simulink model "ANDROID_MODEL"  (R2022b)
settings: Solver=FixedStepAuto  StartTime=0.0  StopTime=inf  RelTol=1e-3
libraries: androiduilib x5, androidcommunicationlib x5, visiongeotforms x3, visionanalysis x1, androidaudiovideolib x1
settings Model: Creator=VIKAS CHEIIURU  LastModifiedBy=VIKAS CHEIIURU
settings SolverCC: PositivePriorityOrder=on
settings OptimizationCC: EnhancedBackFolding=on  PassReuseOutputArgsAs=Individual arguments  ZeroExternalMemoryAtStartup=off  ZeroInternalMemoryAtStartup=off  MaxStackSize=64  OptimizeBlockOrder=speed  DifferentSizesBufferReuse=on  OptimizationCustomize=off  EfficientTunableParamExpr=on
settings DebuggingCC: ParameterTunabilityLossMsg=error
settings HardwareCC: ProdBitPerPointer=32  ProdBitPerSizeT=32  ProdBitPerPtrDiffT=32  ProdLargestAtomicInteger=Long  ProdLargestAtomicFloat=Double  ProdWordSize=32  ProdHWDeviceType=ARM Compatible->ARM Cortex
settings RTWCC: Description=Embedded Coder  SystemTargetFile=ert.tlc  HardwareBoard=Android Device  TLCOptions="-aInlineSetEventsForThisBaseRateFcn=TLC_FALSE -aSuppressMultiTaskScheduler=TLC_FALSE  -aRateBasedStepFcn=0"  TemplateMakefile=ert_default_tmf  RTWVerbose=off  Toolchain=Android SDK/NDK Tools  BuildConfiguration=Faster Runs
settings CodeAppCC: ForceParamTrailComments=on  IgnoreCustomStorageClasses=off  OperatorAnnotations=on  SimulinkDataObjDesc=on  SFDataObjDesc=on  InsertBlockDesc=on
settings ERTTargetCC: SupportVariableSizeSignals=on  ExtModeStaticAlloc=on

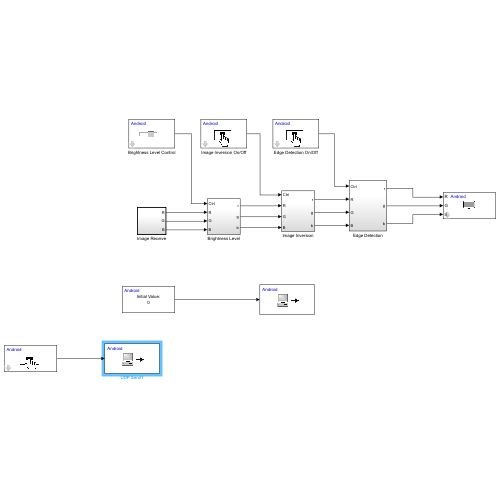
[thumbnail: Simulink's stored preview of the top-level diagram]
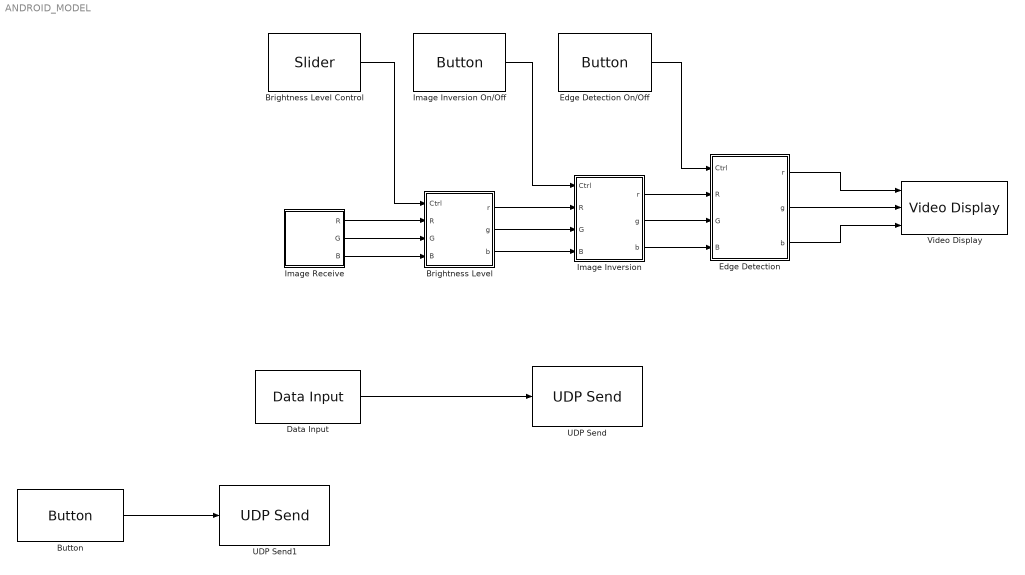
== system ANDROID_MODEL ==
  Brightness Level : Subsystem
  Brightness Level Control : androiduilib/Slider  Min=1  Value=1  Max=4  Resolution=0.1  SliderId=ANDROID_MODEL/Brightness_Level_Control  SampleTime=0.1  BlockPlatform=Android
  Button : androiduilib/Button  ButtonState=Not pressed  ButtonId=ANDROID_MODEL/Button  State=off  SampleTime=0.01  BlockPlatform=Android
  Data Input : androiduilib/Data Input  isCharVector=off  Value=0  CharVector=Hello World  OutputDataType=double  maxCharVectorSize=100  DataInputId=ANDROID_MODEL/Data_Input  SampleTime=0.01
  Edge Detection : Subsystem
  Edge Detection On/Off : androiduilib/Button  ButtonState=Not pressed  ButtonId=ANDROID_MODEL/Edge_Detection_On//Off  State=off  SampleTime=0.1  BlockPlatform=Android
  Image Inversion : Subsystem
  Image Inversion On/Off : androiduilib/Button  ButtonState=Not pressed  ButtonId=ANDROID_MODEL/Image_Inversion_On//Off  State=off  SampleTime=0.1  BlockPlatform=Android
  Image Receive : Subsystem  TreatAsAtomicUnit=on
  UDP Send : androidcommunicationlib/UDP Send  remoteURL='192.168.173.51'  remotePort=26001  localURL='0.0.0.0'  localPortSource=Automatically determine  localPort=-1  sampletime=-1  blockPlatform=Android  separateLengthPort=0
  UDP Send1 : androidcommunicationlib/UDP Send  remoteURL='192.168.173.51'  remotePort=26000  localURL='0.0.0.0'  localPortSource=Automatically determine  localPort=-1  sampletime=-1  blockPlatform=Android  separateLengthPort=0
  Video Display : androidaudiovideolib/Video Display  BlockPlatform=Android
  wires:
  Edge Detection/3(b) -> Video Display/3
  Brightness Level/2(g) -> Image Inversion/3(G)
  Image Inversion/3(b) -> Edge Detection/4(B)
  Image Receive/2(G) -> Brightness Level/3(G)
  Image Inversion On/Off/1 -> Image Inversion/1(Ctrl)
  Edge Detection On/Off/1 -> Edge Detection/1(Ctrl)
  Data Input/1 -> UDP Send/1
  Image Receive/1(R) -> Brightness Level/2(R)
  Image Inversion/2(g) -> Edge Detection/3(G)
  Image Receive/3(B) -> Brightness Level/4(B)
  Brightness Level/1(r) -> Image Inversion/2(R)
  Edge Detection/1(r) -> Video Display/1
  Brightness Level/3(b) -> Image Inversion/4(B)
  Brightness Level Control/1 -> Brightness Level/1(Ctrl)
  Edge Detection/2(g) -> Video Display/2
  Image Inversion/1(r) -> Edge Detection/2(R)
  Button/1 -> UDP Send1/1

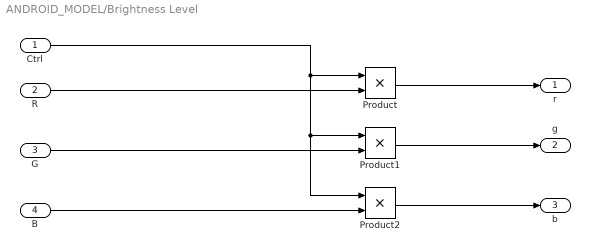
== system ANDROID_MODEL/Brightness Level ==
  Ctrl : Inport
  R : Inport  Port=2
  G : Inport  Port=3
  B : Inport  Port=4
  Product : Product  OutDataTypeStr=uint8  SaturateOnIntegerOverflow=on
  Product1 : Product  OutDataTypeStr=uint8  SaturateOnIntegerOverflow=on
  Product2 : Product  OutDataTypeStr=uint8  SaturateOnIntegerOverflow=on
  r : Outport
  g : Outport  Port=2
  b : Outport  Port=3
  wires:
  R/1 -> Product/2
  Product/1 -> r/1
  G/1 -> Product1/2
  B/1 -> Product2/2
  Product2/1 -> b/1
  Product1/1 -> g/1
  Ctrl/1 -> Product2/1, Product1/1, Product/1

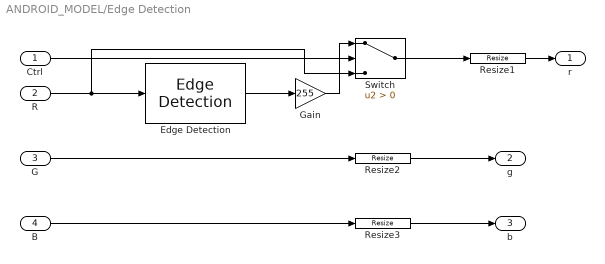
== system ANDROID_MODEL/Edge Detection ==
  Ctrl : Inport
  R : Inport  Port=2
  G : Inport  Port=3
  B : Inport  Port=4
  Edge Detection : visionanalysis/Edge Detection  method=Sobel  outputType=Binary image  userDefinedThreshold=off  thresholdSource=Input port  threshold=20  thresholdTuning=4  edgeThinning=off  threshold_canny=[0.25 0.60]  autoPercent=70  sigma=1  roundingMode=Floor  overflowMode=off  prodOutputMode=Binary point scaling  prodOutputWordLength=32  prodOutputFracLength=8
  Gain : Gain  Gain=255  OutDataTypeStr=uint8
  Resize1 : visiongeotforms/Resize  specify=Output size as a percentage of input size  rfactor=[200 200]  outCols=25  outRows=25  outRowsCols=[25 35]  interp_method=Nearest neighbor  antialias=off  useROI=off  roiFlag=off  roundingMode=Nearest  overflowMode=on  prodOutputMode=Binary point scaling  prodOutputWordLength=32  prodOutputFracLength=10
  Resize2 : visiongeotforms/Resize  specify=Output size as a percentage of input size  rfactor=[200 200]  outCols=25  outRows=25  outRowsCols=[25 35]  interp_method=Nearest neighbor  antialias=off  useROI=off  roiFlag=off  roundingMode=Nearest  overflowMode=on  prodOutputMode=Binary point scaling  prodOutputWordLength=32  prodOutputFracLength=10
  Resize3 : visiongeotforms/Resize  specify=Output size as a percentage of input size  rfactor=[200 200]  outCols=25  outRows=25  outRowsCols=[25 35]  interp_method=Nearest neighbor  antialias=off  useROI=off  roiFlag=off  roundingMode=Nearest  overflowMode=on  prodOutputMode=Binary point scaling  prodOutputWordLength=32  prodOutputFracLength=10
  Switch : Switch  Criteria=u2 > Threshold  SaturateOnIntegerOverflow=off  InputSameDT=off
  r : Outport
  g : Outport  Port=2
  b : Outport  Port=3
  wires:
  Ctrl/1 -> Switch/2
  Edge Detection/1 -> Gain/1
  Gain/1 -> Switch/1
  R/1 -> Switch/3, Edge Detection/1
  Switch/1 -> Resize1/1
  G/1 -> Resize2/1
  B/1 -> Resize3/1
  Resize1/1 -> r/1
  Resize2/1 -> g/1
  Resize3/1 -> b/1

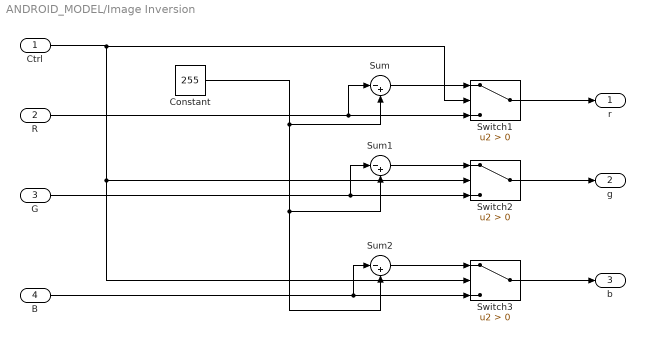
== system ANDROID_MODEL/Image Inversion ==
  Ctrl : Inport
  R : Inport  Port=2
  G : Inport  Port=3
  B : Inport  Port=4
  Constant : Constant  Value=255  OutDataTypeStr=uint8
  Sum : Sum  Inputs=|-+
  Sum1 : Sum  Inputs=|-+
  Sum2 : Sum  Inputs=|-+
  Switch1 : Switch  Criteria=u2 > Threshold  SaturateOnIntegerOverflow=off  InputSameDT=off
  Switch2 : Switch  Criteria=u2 > Threshold  SaturateOnIntegerOverflow=off  InputSameDT=off
  Switch3 : Switch  Criteria=u2 > Threshold  SaturateOnIntegerOverflow=off  InputSameDT=off
  r : Outport
  g : Outport  Port=2
  b : Outport  Port=3
  wires:
  Switch2/1 -> g/1
  Switch1/1 -> r/1
  Constant/1 -> Sum2/2, Sum1/2, Sum/2
  Sum1/1 -> Switch2/1
  Sum/1 -> Switch1/1
  G/1 -> Sum1/1, Switch2/3
  Ctrl/1 -> Switch1/2, Switch3/2, Switch2/2
  Sum2/1 -> Switch3/1
  R/1 -> Sum/1, Switch1/3
  Switch3/1 -> b/1
  B/1 -> Switch3/3, Sum2/1

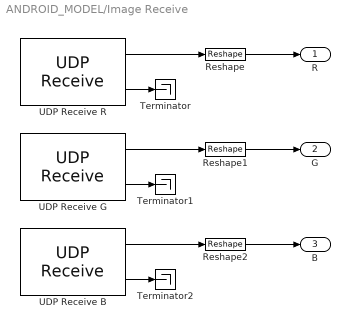
== system ANDROID_MODEL/Image Receive ==
  Reshape : Reshape  OutputDimensionality=Customize  OutputDimensions=[160,120]
  Reshape1 : Reshape  OutputDimensionality=Customize  OutputDimensions=[160,120]
  Reshape2 : Reshape  OutputDimensionality=Customize  OutputDimensions=[160,120]
  Terminator : Terminator
  Terminator1 : Terminator
  Terminator2 : Terminator
  UDP Receive B : androidcommunicationlib/UDP Receive  localURL='0.0.0.0'  localPort=25002  remoteURL='0.0.0.0'  remotePort=-1  recvBufferSize=8192  signalDatatype=uint8  dims=19200  isVarSize=off  showBlockingTime=off  blockingTime=0  sampletime=0.1  blockPlatform=Android
  UDP Receive G : androidcommunicationlib/UDP Receive  localURL='0.0.0.0'  localPort=25001  remoteURL='0.0.0.0'  remotePort=-1  recvBufferSize=8192  signalDatatype=uint8  dims=19200  isVarSize=off  showBlockingTime=off  blockingTime=0  sampletime=0.1  blockPlatform=Android
  UDP Receive R : androidcommunicationlib/UDP Receive  localURL='0.0.0.0'  localPort=25000  remoteURL='0.0.0.0'  remotePort=-1  recvBufferSize=8192  signalDatatype=uint8  dims=19200  isVarSize=off  showBlockingTime=off  blockingTime=0  sampletime=0.1  blockPlatform=Android
  R : Outport
  G : Outport  Port=2
  B : Outport  Port=3
  wires:
  UDP Receive G/1 -> Reshape1/1
  UDP Receive R/1 -> Reshape/1
  UDP Receive B/1 -> Reshape2/1
  UDP Receive G/2 -> Terminator1/1
  UDP Receive B/2 -> Terminator2/1
  UDP Receive R/2 -> Terminator/1
  Reshape/1 -> R/1
  Reshape1/1 -> G/1
  Reshape2/1 -> B/1
